simulink model "c00005M_harness"  (R2018a)
settings: Solver=ode3  StartTime=0.0  StopTime=10.0  RelTol=1e-3  EnableMultiTasking=on
undefined symbols (not defined in the file): b, DiscIntNeverNeededParam, J, K, L, PosMinimaW3, PosMinimaW4, R, sigbuilder_block
(part 3 of 9)

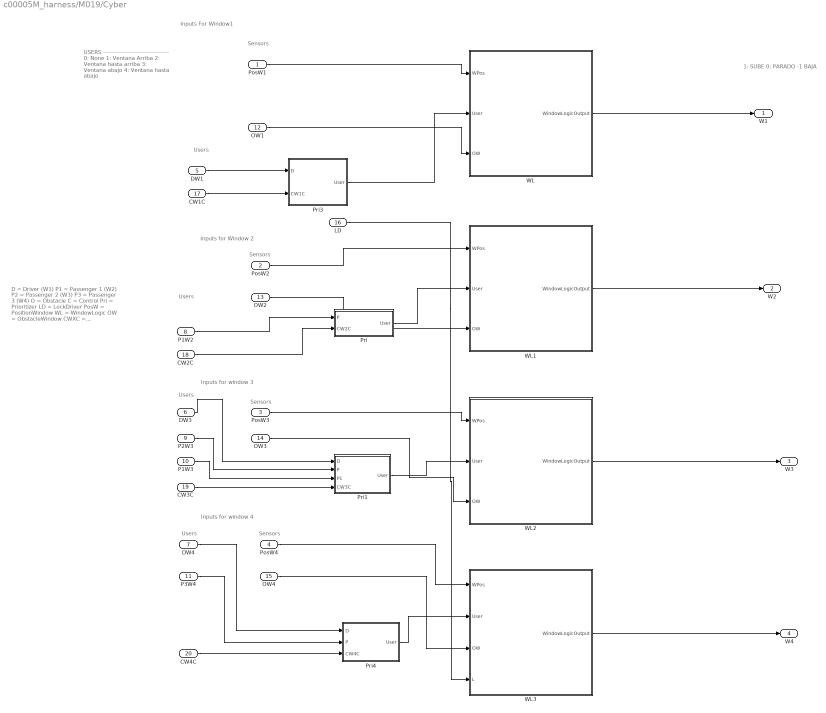
== system c00005M_harness/M019/Cyber ==
  note: Sensors
  note: Inputs For Window1
  note: Inputs for Window 2
  note: Inputs for window 3
  note: Inputs for window 4
  note: Users
  note: Users
  note: Sensors
  note: Users
  note: Sensors
  note: Users
  note: Sensors
  note: USERS
      | ---------------------------------
      | 0: None
      | 1: Ventana Arriba
      | 2: Ventana hasta arriba
      | 3: Ventana abajo
      | 4: Ventana hasta abajo
  note: 1: SUBE
      | 0: PARADO
      | -1 BAJA
  note: D = Driver (W1)
      | P1 = Passenger 1 (W2)
      | P2 = Passenger 2 (W3)
      | P3 = Passenger 3 (W4)
      | O = Obstacle
      | C = Control
      | Pri = Prioritizer
      | LD = LockDriver
      | PosW = PositionWindow
      | WL = WindowLogic
      | OW = ObstacleWindow
      | CWXC = ControlWindowXCentralized
      | S = Sensor
      | L = Lock
      | WPos = WindowPosition
      | M = Memory
      | InW = InputWindow
      | WIn = WindowInput
  PosW1 : Inport
  PosW2 : Inport  Port=2
  PosW3 : Inport  Port=3
  PosW4 : Inport  Port=4
  DW1 : Inport  Port=5
  DW3 : Inport  Port=6
  DW4 : Inport  Port=7
  P1W2 : Inport  Port=8
  P2W3 : Inport  Port=9
  P1W3 : Inport  Port=10
  P3W4 : Inport  Port=11
  OW1 : Inport  Port=12
  OW2 : Inport  Port=13
  OW3 : Inport  Port=14
  OW4 : Inport  Port=15
  LD : Inport  Port=16
  CW1C : Inport  Port=17
  CW2C : Inport  Port=18
  CW3C : Inport  Port=19
  CW4C : Inport  Port=20
  Pri : Subsystem
  Pri1 : Subsystem
  Pri3 : Subsystem
  Pri4 : Subsystem
  WL : Subsystem
  WL1 : Subsystem
  WL2 : Subsystem
  WL3 : Subsystem
  W1 : Outport
  W2 : Outport  Port=2
  W3 : Outport  Port=3
  W4 : Outport  Port=4
  wires:
  CW4C/1 -> Pri4/3(CW4C)
  CW3C/1 -> Pri1/4(CW3C)
  CW2C/1 -> Pri/2(CW2C)
  CW1C/1 -> Pri3/2(CW1C)
  Pri3/1(User) -> WL/2(User)
  WL3/1(WindowLogicOutput) -> W4/1
  WL2/1(WindowLogicOutput) -> W3/1
  Pri4/1(User) -> WL3/2(User)
  OW4/1 -> WL3/3(OW)
  PosW4/1 -> WL3/1(WPos)
  P3W4/1 -> Pri4/2(P)
  DW4/1 -> Pri4/1(D)
  P1W3/1 -> Pri1/3(P1)
  P2W3/1 -> Pri1/2(P)
  DW3/1 -> Pri1/1(D)
  OW3/1 -> WL2/3(OW)
  PosW3/1 -> WL2/1(WPos)
  Pri1/1(User) -> WL2/2(User)
  WL1/1(WindowLogicOutput) -> W2/1
  OW2/1 -> WL1/3(OW)
  PosW2/1 -> WL1/1(WPos)
  P1W2/1 -> Pri/1(P)
  Pri/1(User) -> WL1/2(User)
  WL/1(WindowLogicOutput) -> W1/1
  DW1/1 -> Pri3/1(D)
  OW1/1 -> WL/3(OW)
  PosW1/1 -> WL/1(WPos)
  LD/1 -> WL3/4(L)

== system c00005M_harness/M019/Physical ==
  InW1 : Inport
  InW2 : Inport  Port=2
  InW3 : Inport  Port=3
  InW4 : Inport  Port=4
  W : Subsystem
  W5 : Subsystem
  W6 : Subsystem
  W7 : Subsystem
  W1 : Outport
  W2 : Outport  Port=2
  W3 : Outport  Port=3
  W4 : Outport  Port=4
  wires:
  W7/1(WPos) -> W4/1
  W6/1(WPos) -> W3/1
  W5/1(WPos) -> W2/1
  W/1(WPos) -> W1/1
  InW4/1 -> W7/1(WIn)
  InW3/1 -> W6/1(WIn)
  InW2/1 -> W5/1(WIn)
  InW1/1 -> W/1(WIn)

== system c00005M_harness/M019/S1 ==
  PhyMeasure : Inport
  SensorOut : Outport
  wires:
  PhyMeasure/1 -> SensorOut/1

== system c00005M_harness/M019/S2 ==
  PhyMeasure : Inport
  SensorOut : Outport
  wires:
  PhyMeasure/1 -> SensorOut/1

== system c00005M_harness/M019/S3 ==
  PhyMeasure : Inport
  SensorOut : Outport
  wires:
  PhyMeasure/1 -> SensorOut/1

== system c00005M_harness/M019/S4 ==
  PhyMeasure : Inport
  SensorOut : Outport
  wires:
  PhyMeasure/1 -> SensorOut/1

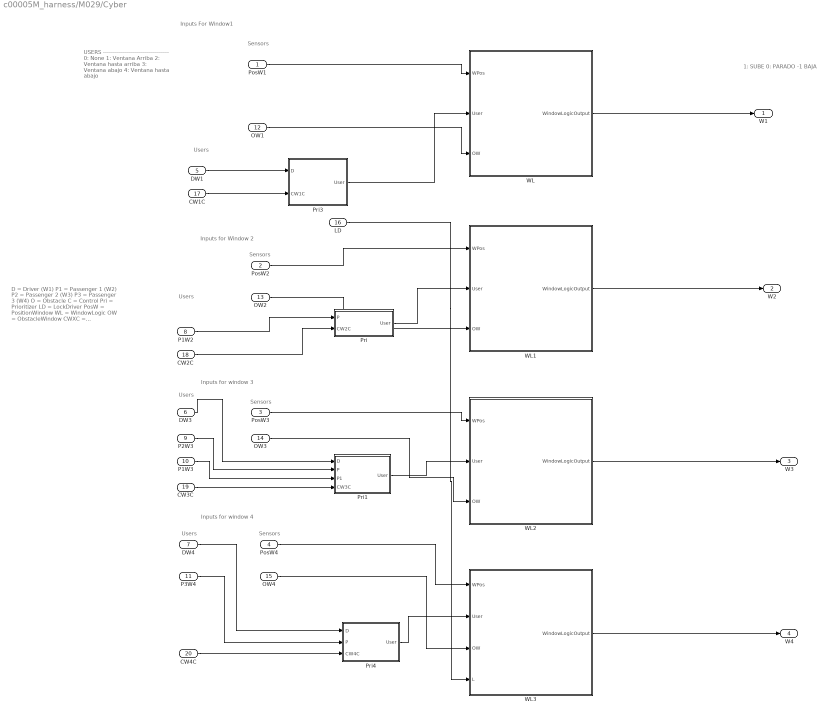
== system c00005M_harness/M029/Cyber ==
  note: Sensors
  note: Inputs For Window1
  note: Inputs for Window 2
  note: Inputs for window 3
  note: Inputs for window 4
  note: Users
  note: Users
  note: Sensors
  note: Users
  note: Sensors
  note: Users
  note: Sensors
  note: USERS
      | ---------------------------------
      | 0: None
      | 1: Ventana Arriba
      | 2: Ventana hasta arriba
      | 3: Ventana abajo
      | 4: Ventana hasta abajo
  note: 1: SUBE
      | 0: PARADO
      | -1 BAJA
  note: D = Driver (W1)
      | P1 = Passenger 1 (W2)
      | P2 = Passenger 2 (W3)
      | P3 = Passenger 3 (W4)
      | O = Obstacle
      | C = Control
      | Pri = Prioritizer
      | LD = LockDriver
      | PosW = PositionWindow
      | WL = WindowLogic
      | OW = ObstacleWindow
      | CWXC = ControlWindowXCentralized
      | S = Sensor
      | L = Lock
      | WPos = WindowPosition
      | M = Memory
      | InW = InputWindow
      | WIn = WindowInput
  PosW1 : Inport
  PosW2 : Inport  Port=2
  PosW3 : Inport  Port=3
  PosW4 : Inport  Port=4
  DW1 : Inport  Port=5
  DW3 : Inport  Port=6
  DW4 : Inport  Port=7
  P1W2 : Inport  Port=8
  P2W3 : Inport  Port=9
  P1W3 : Inport  Port=10
  P3W4 : Inport  Port=11
  OW1 : Inport  Port=12
  OW2 : Inport  Port=13
  OW3 : Inport  Port=14
  OW4 : Inport  Port=15
  LD : Inport  Port=16
  CW1C : Inport  Port=17
  CW2C : Inport  Port=18
  CW3C : Inport  Port=19
  CW4C : Inport  Port=20
  Pri : Subsystem
  Pri1 : Subsystem
  Pri3 : Subsystem
  Pri4 : Subsystem
  WL : Subsystem
  WL1 : Subsystem
  WL2 : Subsystem
  WL3 : Subsystem
  W1 : Outport
  W2 : Outport  Port=2
  W3 : Outport  Port=3
  W4 : Outport  Port=4
  wires:
  CW4C/1 -> Pri4/3(CW4C)
  CW3C/1 -> Pri1/4(CW3C)
  CW2C/1 -> Pri/2(CW2C)
  CW1C/1 -> Pri3/2(CW1C)
  Pri3/1(User) -> WL/2(User)
  WL3/1(WindowLogicOutput) -> W4/1
  WL2/1(WindowLogicOutput) -> W3/1
  Pri4/1(User) -> WL3/2(User)
  OW4/1 -> WL3/3(OW)
  PosW4/1 -> WL3/1(WPos)
  P3W4/1 -> Pri4/2(P)
  DW4/1 -> Pri4/1(D)
  P1W3/1 -> Pri1/3(P1)
  P2W3/1 -> Pri1/2(P)
  DW3/1 -> Pri1/1(D)
  OW3/1 -> WL2/3(OW)
  PosW3/1 -> WL2/1(WPos)
  Pri1/1(User) -> WL2/2(User)
  WL1/1(WindowLogicOutput) -> W2/1
  OW2/1 -> WL1/3(OW)
  PosW2/1 -> WL1/1(WPos)
  P1W2/1 -> Pri/1(P)
  Pri/1(User) -> WL1/2(User)
  WL/1(WindowLogicOutput) -> W1/1
  DW1/1 -> Pri3/1(D)
  OW1/1 -> WL/3(OW)
  PosW1/1 -> WL/1(WPos)
  LD/1 -> WL3/4(L)

== system c00005M_harness/M029/Physical ==
  InW1 : Inport
  InW2 : Inport  Port=2
  InW3 : Inport  Port=3
  InW4 : Inport  Port=4
  W : Subsystem
  W5 : Subsystem
  W6 : Subsystem
  W7 : Subsystem
  W1 : Outport
  W2 : Outport  Port=2
  W3 : Outport  Port=3
  W4 : Outport  Port=4
  wires:
  W7/1(WPos) -> W4/1
  W6/1(WPos) -> W3/1
  W5/1(WPos) -> W2/1
  W/1(WPos) -> W1/1
  InW4/1 -> W7/1(WIn)
  InW3/1 -> W6/1(WIn)
  InW2/1 -> W5/1(WIn)
  InW1/1 -> W/1(WIn)

== system c00005M_harness/M029/S1 ==
  PhyMeasure : Inport
  SensorOut : Outport
  wires:
  PhyMeasure/1 -> SensorOut/1

== system c00005M_harness/M029/S2 ==
  PhyMeasure : Inport
  SensorOut : Outport
  wires:
  PhyMeasure/1 -> SensorOut/1

== system c00005M_harness/M029/S3 ==
  PhyMeasure : Inport
  SensorOut : Outport
  wires:
  PhyMeasure/1 -> SensorOut/1

== system c00005M_harness/M029/S4 ==
  PhyMeasure : Inport
  SensorOut : Outport
  wires:
  PhyMeasure/1 -> SensorOut/1

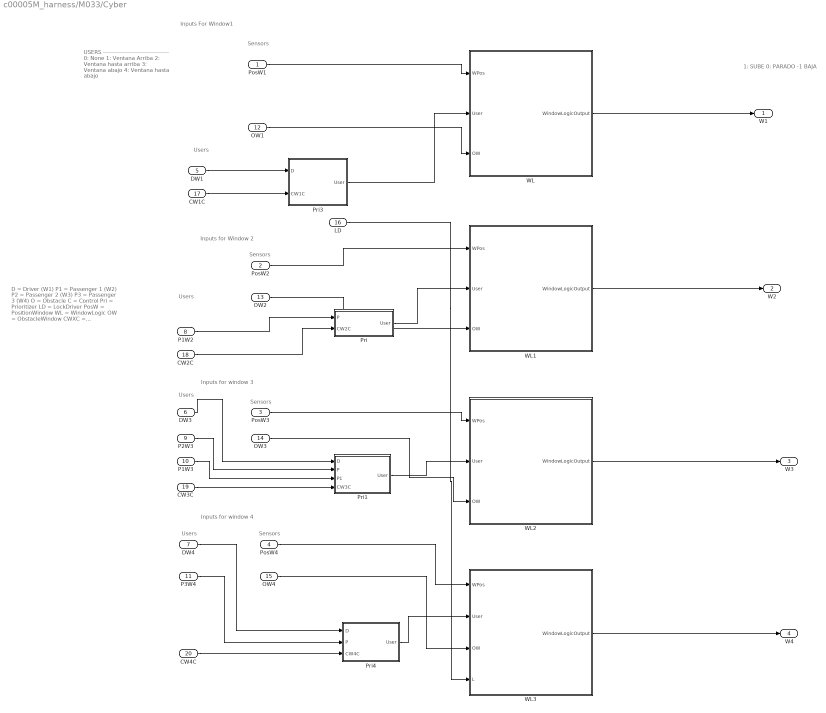
== system c00005M_harness/M033/Cyber ==
  note: Sensors
  note: Inputs For Window1
  note: Inputs for Window 2
  note: Inputs for window 3
  note: Inputs for window 4
  note: Users
  note: Users
  note: Sensors
  note: Users
  note: Sensors
  note: Users
  note: Sensors
  note: USERS
      | ---------------------------------
      | 0: None
      | 1: Ventana Arriba
      | 2: Ventana hasta arriba
      | 3: Ventana abajo
      | 4: Ventana hasta abajo
  note: 1: SUBE
      | 0: PARADO
      | -1 BAJA
  note: D = Driver (W1)
      | P1 = Passenger 1 (W2)
      | P2 = Passenger 2 (W3)
      | P3 = Passenger 3 (W4)
      | O = Obstacle
      | C = Control
      | Pri = Prioritizer
      | LD = LockDriver
      | PosW = PositionWindow
      | WL = WindowLogic
      | OW = ObstacleWindow
      | CWXC = ControlWindowXCentralized
      | S = Sensor
      | L = Lock
      | WPos = WindowPosition
      | M = Memory
      | InW = InputWindow
      | WIn = WindowInput
  PosW1 : Inport
  PosW2 : Inport  Port=2
  PosW3 : Inport  Port=3
  PosW4 : Inport  Port=4
  DW1 : Inport  Port=5
  DW3 : Inport  Port=6
  DW4 : Inport  Port=7
  P1W2 : Inport  Port=8
  P2W3 : Inport  Port=9
  P1W3 : Inport  Port=10
  P3W4 : Inport  Port=11
  OW1 : Inport  Port=12
  OW2 : Inport  Port=13
  OW3 : Inport  Port=14
  OW4 : Inport  Port=15
  LD : Inport  Port=16
  CW1C : Inport  Port=17
  CW2C : Inport  Port=18
  CW3C : Inport  Port=19
  CW4C : Inport  Port=20
  Pri : Subsystem
  Pri1 : Subsystem
  Pri3 : Subsystem
  Pri4 : Subsystem
  WL : Subsystem
  WL1 : Subsystem
  WL2 : Subsystem
  WL3 : Subsystem
  W1 : Outport
  W2 : Outport  Port=2
  W3 : Outport  Port=3
  W4 : Outport  Port=4
  wires:
  CW4C/1 -> Pri4/3(CW4C)
  CW3C/1 -> Pri1/4(CW3C)
  CW2C/1 -> Pri/2(CW2C)
  CW1C/1 -> Pri3/2(CW1C)
  Pri3/1(User) -> WL/2(User)
  WL3/1(WindowLogicOutput) -> W4/1
  WL2/1(WindowLogicOutput) -> W3/1
  Pri4/1(User) -> WL3/2(User)
  OW4/1 -> WL3/3(OW)
  PosW4/1 -> WL3/1(WPos)
  P3W4/1 -> Pri4/2(P)
  DW4/1 -> Pri4/1(D)
  P1W3/1 -> Pri1/3(P1)
  P2W3/1 -> Pri1/2(P)
  DW3/1 -> Pri1/1(D)
  OW3/1 -> WL2/3(OW)
  PosW3/1 -> WL2/1(WPos)
  Pri1/1(User) -> WL2/2(User)
  WL1/1(WindowLogicOutput) -> W2/1
  OW2/1 -> WL1/3(OW)
  PosW2/1 -> WL1/1(WPos)
  P1W2/1 -> Pri/1(P)
  Pri/1(User) -> WL1/2(User)
  WL/1(WindowLogicOutput) -> W1/1
  DW1/1 -> Pri3/1(D)
  OW1/1 -> WL/3(OW)
  PosW1/1 -> WL/1(WPos)
  LD/1 -> WL3/4(L)

== system c00005M_harness/M033/Physical ==
  InW1 : Inport
  InW2 : Inport  Port=2
  InW3 : Inport  Port=3
  InW4 : Inport  Port=4
  W : Subsystem
  W5 : Subsystem
  W6 : Subsystem
  W7 : Subsystem
  W1 : Outport
  W2 : Outport  Port=2
  W3 : Outport  Port=3
  W4 : Outport  Port=4
  wires:
  W7/1(WPos) -> W4/1
  W6/1(WPos) -> W3/1
  W5/1(WPos) -> W2/1
  W/1(WPos) -> W1/1
  InW4/1 -> W7/1(WIn)
  InW3/1 -> W6/1(WIn)
  InW2/1 -> W5/1(WIn)
  InW1/1 -> W/1(WIn)

== system c00005M_harness/M033/S1 ==
  PhyMeasure : Inport
  SensorOut : Outport
  wires:
  PhyMeasure/1 -> SensorOut/1

== system c00005M_harness/M033/S2 ==
  PhyMeasure : Inport
  SensorOut : Outport
  wires:
  PhyMeasure/1 -> SensorOut/1

== system c00005M_harness/M033/S3 ==
  PhyMeasure : Inport
  SensorOut : Outport
  wires:
  PhyMeasure/1 -> SensorOut/1

== system c00005M_harness/M033/S4 ==
  PhyMeasure : Inport
  SensorOut : Outport
  wires:
  PhyMeasure/1 -> SensorOut/1

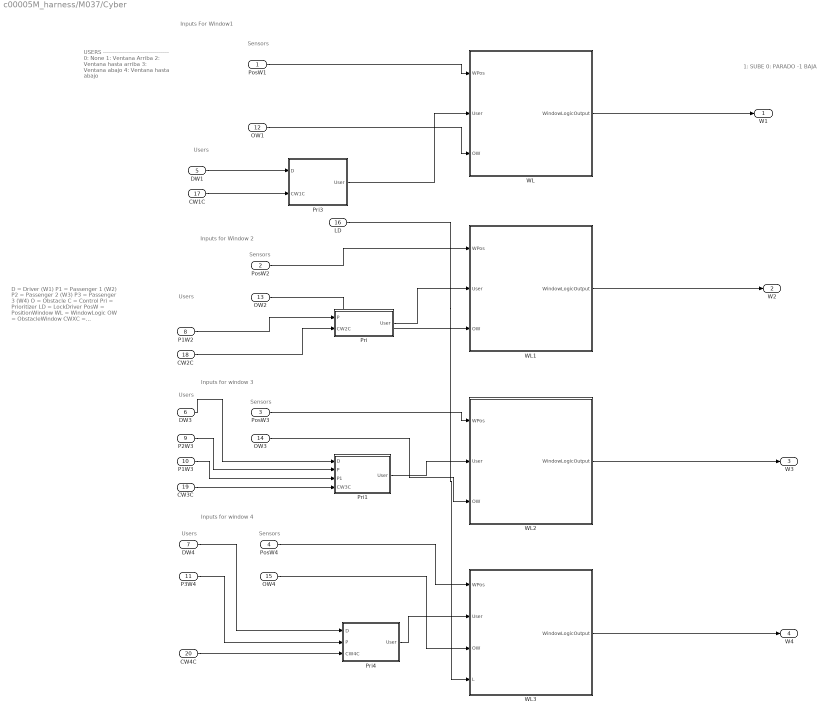
== system c00005M_harness/M037/Cyber ==
  note: Sensors
  note: Inputs For Window1
  note: Inputs for Window 2
  note: Inputs for window 3
  note: Inputs for window 4
  note: Users
  note: Users
  note: Sensors
  note: Users
  note: Sensors
  note: Users
  note: Sensors
  note: USERS
      | ---------------------------------
      | 0: None
      | 1: Ventana Arriba
      | 2: Ventana hasta arriba
      | 3: Ventana abajo
      | 4: Ventana hasta abajo
  note: 1: SUBE
      | 0: PARADO
      | -1 BAJA
  note: D = Driver (W1)
      | P1 = Passenger 1 (W2)
      | P2 = Passenger 2 (W3)
      | P3 = Passenger 3 (W4)
      | O = Obstacle
      | C = Control
      | Pri = Prioritizer
      | LD = LockDriver
      | PosW = PositionWindow
      | WL = WindowLogic
      | OW = ObstacleWindow
      | CWXC = ControlWindowXCentralized
      | S = Sensor
      | L = Lock
      | WPos = WindowPosition
      | M = Memory
      | InW = InputWindow
      | WIn = WindowInput
  PosW1 : Inport
  PosW2 : Inport  Port=2
  PosW3 : Inport  Port=3
  PosW4 : Inport  Port=4
  DW1 : Inport  Port=5
  DW3 : Inport  Port=6
  DW4 : Inport  Port=7
  P1W2 : Inport  Port=8
  P2W3 : Inport  Port=9
  P1W3 : Inport  Port=10
  P3W4 : Inport  Port=11
  OW1 : Inport  Port=12
  OW2 : Inport  Port=13
  OW3 : Inport  Port=14
  OW4 : Inport  Port=15
  LD : Inport  Port=16
  CW1C : Inport  Port=17
  CW2C : Inport  Port=18
  CW3C : Inport  Port=19
  CW4C : Inport  Port=20
  Pri : Subsystem
  Pri1 : Subsystem
  Pri3 : Subsystem
  Pri4 : Subsystem
  WL : Subsystem
  WL1 : Subsystem
  WL2 : Subsystem
  WL3 : Subsystem
  W1 : Outport
  W2 : Outport  Port=2
  W3 : Outport  Port=3
  W4 : Outport  Port=4
  wires:
  CW4C/1 -> Pri4/3(CW4C)
  CW3C/1 -> Pri1/4(CW3C)
  CW2C/1 -> Pri/2(CW2C)
  CW1C/1 -> Pri3/2(CW1C)
  Pri3/1(User) -> WL/2(User)
  WL3/1(WindowLogicOutput) -> W4/1
  WL2/1(WindowLogicOutput) -> W3/1
  Pri4/1(User) -> WL3/2(User)
  OW4/1 -> WL3/3(OW)
  PosW4/1 -> WL3/1(WPos)
  P3W4/1 -> Pri4/2(P)
  DW4/1 -> Pri4/1(D)
  P1W3/1 -> Pri1/3(P1)
  P2W3/1 -> Pri1/2(P)
  DW3/1 -> Pri1/1(D)
  OW3/1 -> WL2/3(OW)
  PosW3/1 -> WL2/1(WPos)
  Pri1/1(User) -> WL2/2(User)
  WL1/1(WindowLogicOutput) -> W2/1
  OW2/1 -> WL1/3(OW)
  PosW2/1 -> WL1/1(WPos)
  P1W2/1 -> Pri/1(P)
  Pri/1(User) -> WL1/2(User)
  WL/1(WindowLogicOutput) -> W1/1
  DW1/1 -> Pri3/1(D)
  OW1/1 -> WL/3(OW)
  PosW1/1 -> WL/1(WPos)
  LD/1 -> WL3/4(L)

== system c00005M_harness/M037/Physical ==
  InW1 : Inport
  InW2 : Inport  Port=2
  InW3 : Inport  Port=3
  InW4 : Inport  Port=4
  W : Subsystem
  W5 : Subsystem
  W6 : Subsystem
  W7 : Subsystem
  W1 : Outport
  W2 : Outport  Port=2
  W3 : Outport  Port=3
  W4 : Outport  Port=4
  wires:
  W7/1(WPos) -> W4/1
  W6/1(WPos) -> W3/1
  W5/1(WPos) -> W2/1
  W/1(WPos) -> W1/1
  InW4/1 -> W7/1(WIn)
  InW3/1 -> W6/1(WIn)
  InW2/1 -> W5/1(WIn)
  InW1/1 -> W/1(WIn)

== system c00005M_harness/M037/S1 ==
  PhyMeasure : Inport
  SensorOut : Outport
  wires:
  PhyMeasure/1 -> SensorOut/1

== system c00005M_harness/M037/S2 ==
  PhyMeasure : Inport
  SensorOut : Outport
  wires:
  PhyMeasure/1 -> SensorOut/1

== system c00005M_harness/M037/S3 ==
  PhyMeasure : Inport
  SensorOut : Outport
  wires:
  PhyMeasure/1 -> SensorOut/1

== system c00005M_harness/M037/S4 ==
  PhyMeasure : Inport
  SensorOut : Outport
  wires:
  PhyMeasure/1 -> SensorOut/1

== system c00005M_harness/M040/Cyber ==
  note: Sensors
  note: Inputs For Window1
  note: Inputs for Window 2
  note: Inputs for window 3
  note: Inputs for window 4
  note: Users
  note: Users
  note: Sensors
  note: Users
  note: Sensors
  note: Users
  note: Sensors
  note: USERS
      | ---------------------------------
      | 0: None
      | 1: Ventana Arriba
      | 2: Ventana hasta arriba
      | 3: Ventana abajo
      | 4: Ventana hasta abajo
  note: 1: SUBE
      | 0: PARADO
      | -1 BAJA
  note: D = Driver (W1)
      | P1 = Passenger 1 (W2)
      | P2 = Passenger 2 (W3)
      | P3 = Passenger 3 (W4)
      | O = Obstacle
      | C = Control
      | Pri = Prioritizer
      | LD = LockDriver
      | PosW = PositionWindow
      | WL = WindowLogic
      | OW = ObstacleWindow
      | CWXC = ControlWindowXCentralized
      | S = Sensor
      | L = Lock
      | WPos = WindowPosition
      | M = Memory
      | InW = InputWindow
      | WIn = WindowInput
  PosW1 : Inport
  PosW2 : Inport  Port=2
  PosW3 : Inport  Port=3
  PosW4 : Inport  Port=4
  DW1 : Inport  Port=5
  DW3 : Inport  Port=6
  DW4 : Inport  Port=7
  P1W2 : Inport  Port=8
  P2W3 : Inport  Port=9
  P1W3 : Inport  Port=10
  P3W4 : Inport  Port=11
  OW1 : Inport  Port=12
  OW2 : Inport  Port=13
  OW3 : Inport  Port=14
  OW4 : Inport  Port=15
  LD : Inport  Port=16
  CW1C : Inport  Port=17
  CW2C : Inport  Port=18
  CW3C : Inport  Port=19
  CW4C : Inport  Port=20
  Pri : Subsystem
  Pri1 : Subsystem
  Pri3 : Subsystem
  Pri4 : Subsystem
  WL : Subsystem
  WL1 : Subsystem
  WL2 : Subsystem
  WL3 : Subsystem
  W1 : Outport
  W2 : Outport  Port=2
  W3 : Outport  Port=3
  W4 : Outport  Port=4
  wires:
  CW4C/1 -> Pri4/3(CW4C)
  CW3C/1 -> Pri1/4(CW3C)
  CW2C/1 -> Pri/2(CW2C)
  CW1C/1 -> Pri3/2(CW1C)
  Pri3/1(User) -> WL/2(User)
  WL3/1(WindowLogicOutput) -> W4/1
  WL2/1(WindowLogicOutput) -> W3/1
  Pri4/1(User) -> WL3/2(User)
  OW4/1 -> WL3/3(OW)
  PosW4/1 -> WL3/1(WPos)
  P3W4/1 -> Pri4/2(P)
  DW4/1 -> Pri4/1(D)
  P1W3/1 -> Pri1/3(P1)
  P2W3/1 -> Pri1/2(P)
  DW3/1 -> Pri1/1(D)
  OW3/1 -> WL2/3(OW)
  PosW3/1 -> WL2/1(WPos)
  Pri1/1(User) -> WL2/2(User)
  WL1/1(WindowLogicOutput) -> W2/1
  OW2/1 -> WL1/3(OW)
  PosW2/1 -> WL1/1(WPos)
  P1W2/1 -> Pri/1(P)
  Pri/1(User) -> WL1/2(User)
  WL/1(WindowLogicOutput) -> W1/1
  DW1/1 -> Pri3/1(D)
  OW1/1 -> WL/3(OW)
  PosW1/1 -> WL/1(WPos)
  LD/1 -> WL3/4(L)

== system c00005M_harness/M040/Physical ==
  InW1 : Inport
  InW2 : Inport  Port=2
  InW3 : Inport  Port=3
  InW4 : Inport  Port=4
  W : Subsystem
  W5 : Subsystem
  W6 : Subsystem
  W7 : Subsystem
  W1 : Outport
  W2 : Outport  Port=2
  W3 : Outport  Port=3
  W4 : Outport  Port=4
  wires:
  W7/1(WPos) -> W4/1
  W6/1(WPos) -> W3/1
  W5/1(WPos) -> W2/1
  W/1(WPos) -> W1/1
  InW4/1 -> W7/1(WIn)
  InW3/1 -> W6/1(WIn)
  InW2/1 -> W5/1(WIn)
  InW1/1 -> W/1(WIn)

== system c00005M_harness/M040/S1 ==
  PhyMeasure : Inport
  SensorOut : Outport
  wires:
  PhyMeasure/1 -> SensorOut/1

== system c00005M_harness/M040/S2 ==
  PhyMeasure : Inport
  SensorOut : Outport
  wires:
  PhyMeasure/1 -> SensorOut/1

== system c00005M_harness/M040/S3 ==
  PhyMeasure : Inport
  SensorOut : Outport
  wires:
  PhyMeasure/1 -> SensorOut/1

== system c00005M_harness/M040/S4 ==
  PhyMeasure : Inport
  SensorOut : Outport
  wires:
  PhyMeasure/1 -> SensorOut/1

== system c00005M_harness/M041/Cyber ==
  note: Sensors
  note: Inputs For Window1
  note: Inputs for Window 2
  note: Inputs for window 3
  note: Inputs for window 4
  note: Users
  note: Users
  note: Sensors
  note: Users
  note: Sensors
  note: Users
  note: Sensors
  note: USERS
      | ---------------------------------
      | 0: None
      | 1: Ventana Arriba
      | 2: Ventana hasta arriba
      | 3: Ventana abajo
      | 4: Ventana hasta abajo
  note: 1: SUBE
      | 0: PARADO
      | -1 BAJA
  note: D = Driver (W1)
      | P1 = Passenger 1 (W2)
      | P2 = Passenger 2 (W3)
      | P3 = Passenger 3 (W4)
      | O = Obstacle
      | C = Control
      | Pri = Prioritizer
      | LD = LockDriver
      | PosW = PositionWindow
      | WL = WindowLogic
      | OW = ObstacleWindow
      | CWXC = ControlWindowXCentralized
      | S = Sensor
      | L = Lock
      | WPos = WindowPosition
      | M = Memory
      | InW = InputWindow
      | WIn = WindowInput
  PosW1 : Inport
  PosW2 : Inport  Port=2
  PosW3 : Inport  Port=3
  PosW4 : Inport  Port=4
  DW1 : Inport  Port=5
  DW3 : Inport  Port=6
  DW4 : Inport  Port=7
  P1W2 : Inport  Port=8
  P2W3 : Inport  Port=9
  P1W3 : Inport  Port=10
  P3W4 : Inport  Port=11
  OW1 : Inport  Port=12
  OW2 : Inport  Port=13
  OW3 : Inport  Port=14
  OW4 : Inport  Port=15
  LD : Inport  Port=16
  CW1C : Inport  Port=17
  CW2C : Inport  Port=18
  CW3C : Inport  Port=19
  CW4C : Inport  Port=20
  Pri : Subsystem
  Pri1 : Subsystem
  Pri3 : Subsystem
  Pri4 : Subsystem
  WL : Subsystem
  WL1 : Subsystem
  WL2 : Subsystem
  WL3 : Subsystem
  W1 : Outport
  W2 : Outport  Port=2
  W3 : Outport  Port=3
  W4 : Outport  Port=4
  wires:
  CW4C/1 -> Pri4/3(CW4C)
  CW3C/1 -> Pri1/4(CW3C)
  CW2C/1 -> Pri/2(CW2C)
  CW1C/1 -> Pri3/2(CW1C)
  Pri3/1(User) -> WL/2(User)
  WL3/1(WindowLogicOutput) -> W4/1
  WL2/1(WindowLogicOutput) -> W3/1
  Pri4/1(User) -> WL3/2(User)
  OW4/1 -> WL3/3(OW)
  PosW4/1 -> WL3/1(WPos)
  P3W4/1 -> Pri4/2(P)
  DW4/1 -> Pri4/1(D)
  P1W3/1 -> Pri1/3(P1)
  P2W3/1 -> Pri1/2(P)
  DW3/1 -> Pri1/1(D)
  OW3/1 -> WL2/3(OW)
  PosW3/1 -> WL2/1(WPos)
  Pri1/1(User) -> WL2/2(User)
  WL1/1(WindowLogicOutput) -> W2/1
  OW2/1 -> WL1/3(OW)
  PosW2/1 -> WL1/1(WPos)
  P1W2/1 -> Pri/1(P)
  Pri/1(User) -> WL1/2(User)
  WL/1(WindowLogicOutput) -> W1/1
  DW1/1 -> Pri3/1(D)
  OW1/1 -> WL/3(OW)
  PosW1/1 -> WL/1(WPos)
  LD/1 -> WL3/4(L)

== system c00005M_harness/M041/Physical ==
  InW1 : Inport
  InW2 : Inport  Port=2
  InW3 : Inport  Port=3
  InW4 : Inport  Port=4
  W : Subsystem
  W5 : Subsystem
  W6 : Subsystem
  W7 : Subsystem
  W1 : Outport
  W2 : Outport  Port=2
  W3 : Outport  Port=3
  W4 : Outport  Port=4
  wires:
  W7/1(WPos) -> W4/1
  W6/1(WPos) -> W3/1
  W5/1(WPos) -> W2/1
  W/1(WPos) -> W1/1
  InW4/1 -> W7/1(WIn)
  InW3/1 -> W6/1(WIn)
  InW2/1 -> W5/1(WIn)
  InW1/1 -> W/1(WIn)

== system c00005M_harness/M041/S1 ==
  PhyMeasure : Inport
  SensorOut : Outport
  wires:
  PhyMeasure/1 -> SensorOut/1

== system c00005M_harness/M041/S2 ==
  PhyMeasure : Inport
  SensorOut : Outport
  wires:
  PhyMeasure/1 -> SensorOut/1

== system c00005M_harness/M041/S3 ==
  PhyMeasure : Inport
  SensorOut : Outport
  wires:
  PhyMeasure/1 -> SensorOut/1

== system c00005M_harness/M041/S4 ==
  PhyMeasure : Inport
  SensorOut : Outport
  wires:
  PhyMeasure/1 -> SensorOut/1

== system c00005M_harness/M043/Cyber ==
  note: Sensors
  note: Inputs For Window1
  note: Inputs for Window 2
  note: Inputs for window 3
  note: Inputs for window 4
  note: Users
  note: Users
  note: Sensors
  note: Users
  note: Sensors
  note: Users
  note: Sensors
  note: USERS
      | ---------------------------------
      | 0: None
      | 1: Ventana Arriba
      | 2: Ventana hasta arriba
      | 3: Ventana abajo
      | 4: Ventana hasta abajo
  note: 1: SUBE
      | 0: PARADO
      | -1 BAJA
  note: D = Driver (W1)
      | P1 = Passenger 1 (W2)
      | P2 = Passenger 2 (W3)
      | P3 = Passenger 3 (W4)
      | O = Obstacle
      | C = Control
      | Pri = Prioritizer
      | LD = LockDriver
      | PosW = PositionWindow
      | WL = WindowLogic
      | OW = ObstacleWindow
      | CWXC = ControlWindowXCentralized
      | S = Sensor
      | L = Lock
      | WPos = WindowPosition
      | M = Memory
      | InW = InputWindow
      | WIn = WindowInput
  PosW1 : Inport
  PosW2 : Inport  Port=2
  PosW3 : Inport  Port=3
  PosW4 : Inport  Port=4
  DW1 : Inport  Port=5
  DW3 : Inport  Port=6
  DW4 : Inport  Port=7
  P1W2 : Inport  Port=8
  P2W3 : Inport  Port=9
  P1W3 : Inport  Port=10
  P3W4 : Inport  Port=11
  OW1 : Inport  Port=12
  OW2 : Inport  Port=13
  OW3 : Inport  Port=14
  OW4 : Inport  Port=15
  LD : Inport  Port=16
  CW1C : Inport  Port=17
  CW2C : Inport  Port=18
  CW3C : Inport  Port=19
  CW4C : Inport  Port=20
  Pri : Subsystem
  Pri1 : Subsystem
  Pri3 : Subsystem
  Pri4 : Subsystem
  WL : Subsystem
  WL1 : Subsystem
  WL2 : Subsystem
  WL3 : Subsystem
  W1 : Outport
  W2 : Outport  Port=2
  W3 : Outport  Port=3
  W4 : Outport  Port=4
  wires:
  CW4C/1 -> Pri4/3(CW4C)
  CW3C/1 -> Pri1/4(CW3C)
  CW2C/1 -> Pri/2(CW2C)
  CW1C/1 -> Pri3/2(CW1C)
  Pri3/1(User) -> WL/2(User)
  WL3/1(WindowLogicOutput) -> W4/1
  WL2/1(WindowLogicOutput) -> W3/1
  Pri4/1(User) -> WL3/2(User)
  OW4/1 -> WL3/3(OW)
  PosW4/1 -> WL3/1(WPos)
  P3W4/1 -> Pri4/2(P)
  DW4/1 -> Pri4/1(D)
  P1W3/1 -> Pri1/3(P1)
  P2W3/1 -> Pri1/2(P)
  DW3/1 -> Pri1/1(D)
  OW3/1 -> WL2/3(OW)
  PosW3/1 -> WL2/1(WPos)
  Pri1/1(User) -> WL2/2(User)
  WL1/1(WindowLogicOutput) -> W2/1
  OW2/1 -> WL1/3(OW)
  PosW2/1 -> WL1/1(WPos)
  P1W2/1 -> Pri/1(P)
  Pri/1(User) -> WL1/2(User)
  WL/1(WindowLogicOutput) -> W1/1
  DW1/1 -> Pri3/1(D)
  OW1/1 -> WL/3(OW)
  PosW1/1 -> WL/1(WPos)
  LD/1 -> WL3/4(L)

== system c00005M_harness/M043/Physical ==
  InW1 : Inport
  InW2 : Inport  Port=2
  InW3 : Inport  Port=3
  InW4 : Inport  Port=4
  W : Subsystem
  W5 : Subsystem
  W6 : Subsystem
  W7 : Subsystem
  W1 : Outport
  W2 : Outport  Port=2
  W3 : Outport  Port=3
  W4 : Outport  Port=4
  wires:
  W7/1(WPos) -> W4/1
  W6/1(WPos) -> W3/1
  W5/1(WPos) -> W2/1
  W/1(WPos) -> W1/1
  InW4/1 -> W7/1(WIn)
  InW3/1 -> W6/1(WIn)
  InW2/1 -> W5/1(WIn)
  InW1/1 -> W/1(WIn)

== system c00005M_harness/M043/S1 ==
  PhyMeasure : Inport
  SensorOut : Outport
  wires:
  PhyMeasure/1 -> SensorOut/1

== system c00005M_harness/M043/S2 ==
  PhyMeasure : Inport
  SensorOut : Outport
  wires:
  PhyMeasure/1 -> SensorOut/1

== system c00005M_harness/M043/S3 ==
  PhyMeasure : Inport
  SensorOut : Outport
  wires:
  PhyMeasure/1 -> SensorOut/1

== system c00005M_harness/M043/S4 ==
  PhyMeasure : Inport
  SensorOut : Outport
  wires:
  PhyMeasure/1 -> SensorOut/1

== system c00005M_harness/M046/Cyber ==
  note: Sensors
  note: Inputs For Window1
  note: Inputs for Window 2
  note: Inputs for window 3
  note: Inputs for window 4
  note: Users
  note: Users
  note: Sensors
  note: Users
  note: Sensors
  note: Users
  note: Sensors
  note: USERS
      | ---------------------------------
      | 0: None
      | 1: Ventana Arriba
      | 2: Ventana hasta arriba
      | 3: Ventana abajo
      | 4: Ventana hasta abajo
  note: 1: SUBE
      | 0: PARADO
      | -1 BAJA
  note: D = Driver (W1)
      | P1 = Passenger 1 (W2)
      | P2 = Passenger 2 (W3)
      | P3 = Passenger 3 (W4)
      | O = Obstacle
      | C = Control
      | Pri = Prioritizer
      | LD = LockDriver
      | PosW = PositionWindow
      | WL = WindowLogic
      | OW = ObstacleWindow
      | CWXC = ControlWindowXCentralized
      | S = Sensor
      | L = Lock
      | WPos = WindowPosition
      | M = Memory
      | InW = InputWindow
      | WIn = WindowInput
  PosW1 : Inport
  PosW2 : Inport  Port=2
  PosW3 : Inport  Port=3
  PosW4 : Inport  Port=4
  DW1 : Inport  Port=5
  DW3 : Inport  Port=6
  DW4 : Inport  Port=7
  P1W2 : Inport  Port=8
  P2W3 : Inport  Port=9
  P1W3 : Inport  Port=10
  P3W4 : Inport  Port=11
  OW1 : Inport  Port=12
  OW2 : Inport  Port=13
  OW3 : Inport  Port=14
  OW4 : Inport  Port=15
  LD : Inport  Port=16
  CW1C : Inport  Port=17
  CW2C : Inport  Port=18
  CW3C : Inport  Port=19
  CW4C : Inport  Port=20
  Pri : Subsystem
  Pri1 : Subsystem
  Pri3 : Subsystem
  Pri4 : Subsystem
  WL : Subsystem
  WL1 : Subsystem
  WL2 : Subsystem
  WL3 : Subsystem
  W1 : Outport
  W2 : Outport  Port=2
  W3 : Outport  Port=3
  W4 : Outport  Port=4
  wires:
  CW4C/1 -> Pri4/3(CW4C)
  CW3C/1 -> Pri1/4(CW3C)
  CW2C/1 -> Pri/2(CW2C)
  CW1C/1 -> Pri3/2(CW1C)
  Pri3/1(User) -> WL/2(User)
  WL3/1(WindowLogicOutput) -> W4/1
  WL2/1(WindowLogicOutput) -> W3/1
  Pri4/1(User) -> WL3/2(User)
  OW4/1 -> WL3/3(OW)
  PosW4/1 -> WL3/1(WPos)
  P3W4/1 -> Pri4/2(P)
  DW4/1 -> Pri4/1(D)
  P1W3/1 -> Pri1/3(P1)
  P2W3/1 -> Pri1/2(P)
  DW3/1 -> Pri1/1(D)
  OW3/1 -> WL2/3(OW)
  PosW3/1 -> WL2/1(WPos)
  Pri1/1(User) -> WL2/2(User)
  WL1/1(WindowLogicOutput) -> W2/1
  OW2/1 -> WL1/3(OW)
  PosW2/1 -> WL1/1(WPos)
  P1W2/1 -> Pri/1(P)
  Pri/1(User) -> WL1/2(User)
  WL/1(WindowLogicOutput) -> W1/1
  DW1/1 -> Pri3/1(D)
  OW1/1 -> WL/3(OW)
  PosW1/1 -> WL/1(WPos)
  LD/1 -> WL3/4(L)

== system c00005M_harness/M046/Physical ==
  InW1 : Inport
  InW2 : Inport  Port=2
  InW3 : Inport  Port=3
  InW4 : Inport  Port=4
  W : Subsystem
  W5 : Subsystem
  W6 : Subsystem
  W7 : Subsystem
  W1 : Outport
  W2 : Outport  Port=2
  W3 : Outport  Port=3
  W4 : Outport  Port=4
  wires:
  W7/1(WPos) -> W4/1
  W6/1(WPos) -> W3/1
  W5/1(WPos) -> W2/1
  W/1(WPos) -> W1/1
  InW4/1 -> W7/1(WIn)
  InW3/1 -> W6/1(WIn)
  InW2/1 -> W5/1(WIn)
  InW1/1 -> W/1(WIn)

== system c00005M_harness/M046/S1 ==
  PhyMeasure : Inport
  SensorOut : Outport
  wires:
  PhyMeasure/1 -> SensorOut/1

== system c00005M_harness/M046/S2 ==
  PhyMeasure : Inport
  SensorOut : Outport
  wires:
  PhyMeasure/1 -> SensorOut/1

== system c00005M_harness/M046/S3 ==
  PhyMeasure : Inport
  SensorOut : Outport
  wires:
  PhyMeasure/1 -> SensorOut/1

== system c00005M_harness/M046/S4 ==
  PhyMeasure : Inport
  SensorOut : Outport
  wires:
  PhyMeasure/1 -> SensorOut/1

== system c00005M_harness/M048/Cyber ==
  note: Sensors
  note: Inputs For Window1
  note: Inputs for Window 2
  note: Inputs for window 3
  note: Inputs for window 4
  note: Users
  note: Users
  note: Sensors
  note: Users
  note: Sensors
  note: Users
  note: Sensors
  note: USERS
      | ---------------------------------
      | 0: None
      | 1: Ventana Arriba
      | 2: Ventana hasta arriba
      | 3: Ventana abajo
      | 4: Ventana hasta abajo
  note: 1: SUBE
      | 0: PARADO
      | -1 BAJA
  note: D = Driver (W1)
      | P1 = Passenger 1 (W2)
      | P2 = Passenger 2 (W3)
      | P3 = Passenger 3 (W4)
      | O = Obstacle
      | C = Control
      | Pri = Prioritizer
      | LD = LockDriver
      | PosW = PositionWindow
      | WL = WindowLogic
      | OW = ObstacleWindow
      | CWXC = ControlWindowXCentralized
      | S = Sensor
      | L = Lock
      | WPos = WindowPosition
      | M = Memory
      | InW = InputWindow
      | WIn = WindowInput
  PosW1 : Inport
  PosW2 : Inport  Port=2
  PosW3 : Inport  Port=3
  PosW4 : Inport  Port=4
  DW1 : Inport  Port=5
  DW3 : Inport  Port=6
  DW4 : Inport  Port=7
  P1W2 : Inport  Port=8
  P2W3 : Inport  Port=9
  P1W3 : Inport  Port=10
  P3W4 : Inport  Port=11
  OW1 : Inport  Port=12
  OW2 : Inport  Port=13
  OW3 : Inport  Port=14
  OW4 : Inport  Port=15
  LD : Inport  Port=16
  CW1C : Inport  Port=17
  CW2C : Inport  Port=18
  CW3C : Inport  Port=19
  CW4C : Inport  Port=20
  Pri : Subsystem
  Pri1 : Subsystem
  Pri3 : Subsystem
  Pri4 : Subsystem
  WL : Subsystem
  WL1 : Subsystem
  WL2 : Subsystem
  WL3 : Subsystem
  W1 : Outport
  W2 : Outport  Port=2
  W3 : Outport  Port=3
  W4 : Outport  Port=4
  wires:
  CW4C/1 -> Pri4/3(CW4C)
  CW3C/1 -> Pri1/4(CW3C)
  CW2C/1 -> Pri/2(CW2C)
  CW1C/1 -> Pri3/2(CW1C)
  Pri3/1(User) -> WL/2(User)
  WL3/1(WindowLogicOutput) -> W4/1
  WL2/1(WindowLogicOutput) -> W3/1
  Pri4/1(User) -> WL3/2(User)
  OW4/1 -> WL3/3(OW)
  PosW4/1 -> WL3/1(WPos)
  P3W4/1 -> Pri4/2(P)
  DW4/1 -> Pri4/1(D)
  P1W3/1 -> Pri1/3(P1)
  P2W3/1 -> Pri1/2(P)
  DW3/1 -> Pri1/1(D)
  OW3/1 -> WL2/3(OW)
  PosW3/1 -> WL2/1(WPos)
  Pri1/1(User) -> WL2/2(User)
  WL1/1(WindowLogicOutput) -> W2/1
  OW2/1 -> WL1/3(OW)
  PosW2/1 -> WL1/1(WPos)
  P1W2/1 -> Pri/1(P)
  Pri/1(User) -> WL1/2(User)
  WL/1(WindowLogicOutput) -> W1/1
  DW1/1 -> Pri3/1(D)
  OW1/1 -> WL/3(OW)
  PosW1/1 -> WL/1(WPos)
  LD/1 -> WL3/4(L)

== system c00005M_harness/M048/Physical ==
  InW1 : Inport
  InW2 : Inport  Port=2
  InW3 : Inport  Port=3
  InW4 : Inport  Port=4
  W : Subsystem
  W5 : Subsystem
  W6 : Subsystem
  W7 : Subsystem
  W1 : Outport
  W2 : Outport  Port=2
  W3 : Outport  Port=3
  W4 : Outport  Port=4
  wires:
  W7/1(WPos) -> W4/1
  W6/1(WPos) -> W3/1
  W5/1(WPos) -> W2/1
  W/1(WPos) -> W1/1
  InW4/1 -> W7/1(WIn)
  InW3/1 -> W6/1(WIn)
  InW2/1 -> W5/1(WIn)
  InW1/1 -> W/1(WIn)

== system c00005M_harness/M048/S1 ==
  PhyMeasure : Inport
  SensorOut : Outport
  wires:
  PhyMeasure/1 -> SensorOut/1

== system c00005M_harness/M048/S2 ==
  PhyMeasure : Inport
  SensorOut : Outport
  wires:
  PhyMeasure/1 -> SensorOut/1

== system c00005M_harness/M048/S3 ==
  PhyMeasure : Inport
  SensorOut : Outport
  wires:
  PhyMeasure/1 -> SensorOut/1

== system c00005M_harness/M048/S4 ==
  PhyMeasure : Inport
  SensorOut : Outport
  wires:
  PhyMeasure/1 -> SensorOut/1

== system c00005M_harness/M057/Cyber ==
  note: Sensors
  note: Inputs For Window1
  note: Inputs for Window 2
  note: Inputs for window 3
  note: Inputs for window 4
  note: Users
  note: Users
  note: Sensors
  note: Users
  note: Sensors
  note: Users
  note: Sensors
  note: USERS
      | ---------------------------------
      | 0: None
      | 1: Ventana Arriba
      | 2: Ventana hasta arriba
      | 3: Ventana abajo
      | 4: Ventana hasta abajo
  note: 1: SUBE
      | 0: PARADO
      | -1 BAJA
  note: D = Driver (W1)
      | P1 = Passenger 1 (W2)
      | P2 = Passenger 2 (W3)
      | P3 = Passenger 3 (W4)
      | O = Obstacle
      | C = Control
      | Pri = Prioritizer
      | LD = LockDriver
      | PosW = PositionWindow
      | WL = WindowLogic
      | OW = ObstacleWindow
      | CWXC = ControlWindowXCentralized
      | S = Sensor
      | L = Lock
      | WPos = WindowPosition
      | M = Memory
      | InW = InputWindow
      | WIn = WindowInput
  PosW1 : Inport
  PosW2 : Inport  Port=2
  PosW3 : Inport  Port=3
  PosW4 : Inport  Port=4
  DW1 : Inport  Port=5
  DW3 : Inport  Port=6
  DW4 : Inport  Port=7
  P1W2 : Inport  Port=8
  P2W3 : Inport  Port=9
  P1W3 : Inport  Port=10
  P3W4 : Inport  Port=11
  OW1 : Inport  Port=12
  OW2 : Inport  Port=13
  OW3 : Inport  Port=14
  OW4 : Inport  Port=15
  LD : Inport  Port=16
  CW1C : Inport  Port=17
  CW2C : Inport  Port=18
  CW3C : Inport  Port=19
  CW4C : Inport  Port=20
  Pri : Subsystem
  Pri1 : Subsystem
  Pri3 : Subsystem
  Pri4 : Subsystem
  WL : Subsystem
  WL1 : Subsystem
  WL2 : Subsystem
  WL3 : Subsystem
  W1 : Outport
  W2 : Outport  Port=2
  W3 : Outport  Port=3
  W4 : Outport  Port=4
  wires:
  CW4C/1 -> Pri4/3(CW4C)
  CW3C/1 -> Pri1/4(CW3C)
  CW2C/1 -> Pri/2(CW2C)
  CW1C/1 -> Pri3/2(CW1C)
  Pri3/1(User) -> WL/2(User)
  WL3/1(WindowLogicOutput) -> W4/1
  WL2/1(WindowLogicOutput) -> W3/1
  Pri4/1(User) -> WL3/2(User)
  OW4/1 -> WL3/3(OW)
  PosW4/1 -> WL3/1(WPos)
  P3W4/1 -> Pri4/2(P)
  DW4/1 -> Pri4/1(D)
  P1W3/1 -> Pri1/3(P1)
  P2W3/1 -> Pri1/2(P)
  DW3/1 -> Pri1/1(D)
  OW3/1 -> WL2/3(OW)
  PosW3/1 -> WL2/1(WPos)
  Pri1/1(User) -> WL2/2(User)
  WL1/1(WindowLogicOutput) -> W2/1
  OW2/1 -> WL1/3(OW)
  PosW2/1 -> WL1/1(WPos)
  P1W2/1 -> Pri/1(P)
  Pri/1(User) -> WL1/2(User)
  WL/1(WindowLogicOutput) -> W1/1
  DW1/1 -> Pri3/1(D)
  OW1/1 -> WL/3(OW)
  PosW1/1 -> WL/1(WPos)
  LD/1 -> WL3/4(L)

== system c00005M_harness/M057/Physical ==
  InW1 : Inport
  InW2 : Inport  Port=2
  InW3 : Inport  Port=3
  InW4 : Inport  Port=4
  W : Subsystem
  W5 : Subsystem
  W6 : Subsystem
  W7 : Subsystem
  W1 : Outport
  W2 : Outport  Port=2
  W3 : Outport  Port=3
  W4 : Outport  Port=4
  wires:
  W7/1(WPos) -> W4/1
  W6/1(WPos) -> W3/1
  W5/1(WPos) -> W2/1
  W/1(WPos) -> W1/1
  InW4/1 -> W7/1(WIn)
  InW3/1 -> W6/1(WIn)
  InW2/1 -> W5/1(WIn)
  InW1/1 -> W/1(WIn)

== system c00005M_harness/M057/S1 ==
  PhyMeasure : Inport
  SensorOut : Outport
  wires:
  PhyMeasure/1 -> SensorOut/1

== system c00005M_harness/M057/S2 ==
  PhyMeasure : Inport
  SensorOut : Outport
  wires:
  PhyMeasure/1 -> SensorOut/1

== system c00005M_harness/M057/S3 ==
  PhyMeasure : Inport
  SensorOut : Outport
  wires:
  PhyMeasure/1 -> SensorOut/1

== system c00005M_harness/M057/S4 ==
  PhyMeasure : Inport
  SensorOut : Outport
  wires:
  PhyMeasure/1 -> SensorOut/1

== system c00005M_harness/M058/Cyber ==
  note: Sensors
  note: Inputs For Window1
  note: Inputs for Window 2
  note: Inputs for window 3
  note: Inputs for window 4
  note: Users
  note: Users
  note: Sensors
  note: Users
  note: Sensors
  note: Users
  note: Sensors
  note: USERS
      | ---------------------------------
      | 0: None
      | 1: Ventana Arriba
      | 2: Ventana hasta arriba
      | 3: Ventana abajo
      | 4: Ventana hasta abajo
  note: 1: SUBE
      | 0: PARADO
      | -1 BAJA
  note: D = Driver (W1)
      | P1 = Passenger 1 (W2)
      | P2 = Passenger 2 (W3)
      | P3 = Passenger 3 (W4)
      | O = Obstacle
      | C = Control
      | Pri = Prioritizer
      | LD = LockDriver
      | PosW = PositionWindow
      | WL = WindowLogic
      | OW = ObstacleWindow
      | CWXC = ControlWindowXCentralized
      | S = Sensor
      | L = Lock
      | WPos = WindowPosition
      | M = Memory
      | InW = InputWindow
      | WIn = WindowInput
  PosW1 : Inport
  PosW2 : Inport  Port=2
  PosW3 : Inport  Port=3
  PosW4 : Inport  Port=4
  DW1 : Inport  Port=5
  DW3 : Inport  Port=6
  DW4 : Inport  Port=7
  P1W2 : Inport  Port=8
  P2W3 : Inport  Port=9
  P1W3 : Inport  Port=10
  P3W4 : Inport  Port=11
  OW1 : Inport  Port=12
  OW2 : Inport  Port=13
  OW3 : Inport  Port=14
  OW4 : Inport  Port=15
  LD : Inport  Port=16
  CW1C : Inport  Port=17
  CW2C : Inport  Port=18
  CW3C : Inport  Port=19
  CW4C : Inport  Port=20
  Pri : Subsystem
  Pri1 : Subsystem
  Pri3 : Subsystem
  Pri4 : Subsystem
  WL : Subsystem
  WL1 : Subsystem
  WL2 : Subsystem
  WL3 : Subsystem
  W1 : Outport
  W2 : Outport  Port=2
  W3 : Outport  Port=3
  W4 : Outport  Port=4
  wires:
  CW4C/1 -> Pri4/3(CW4C)
  CW3C/1 -> Pri1/4(CW3C)
  CW2C/1 -> Pri/2(CW2C)
  CW1C/1 -> Pri3/2(CW1C)
  Pri3/1(User) -> WL/2(User)
  WL3/1(WindowLogicOutput) -> W4/1
  WL2/1(WindowLogicOutput) -> W3/1
  Pri4/1(User) -> WL3/2(User)
  OW4/1 -> WL3/3(OW)
  PosW4/1 -> WL3/1(WPos)
  P3W4/1 -> Pri4/2(P)
  DW4/1 -> Pri4/1(D)
  P1W3/1 -> Pri1/3(P1)
  P2W3/1 -> Pri1/2(P)
  DW3/1 -> Pri1/1(D)
  OW3/1 -> WL2/3(OW)
  PosW3/1 -> WL2/1(WPos)
  Pri1/1(User) -> WL2/2(User)
  WL1/1(WindowLogicOutput) -> W2/1
  OW2/1 -> WL1/3(OW)
  PosW2/1 -> WL1/1(WPos)
  P1W2/1 -> Pri/1(P)
  Pri/1(User) -> WL1/2(User)
  WL/1(WindowLogicOutput) -> W1/1
  DW1/1 -> Pri3/1(D)
  OW1/1 -> WL/3(OW)
  PosW1/1 -> WL/1(WPos)
  LD/1 -> WL3/4(L)

== system c00005M_harness/M058/Physical ==
  InW1 : Inport
  InW2 : Inport  Port=2
  InW3 : Inport  Port=3
  InW4 : Inport  Port=4
  W : Subsystem
  W5 : Subsystem
  W6 : Subsystem
  W7 : Subsystem
  W1 : Outport
  W2 : Outport  Port=2
  W3 : Outport  Port=3
  W4 : Outport  Port=4
  wires:
  W7/1(WPos) -> W4/1
  W6/1(WPos) -> W3/1
  W5/1(WPos) -> W2/1
  W/1(WPos) -> W1/1
  InW4/1 -> W7/1(WIn)
  InW3/1 -> W6/1(WIn)
  InW2/1 -> W5/1(WIn)
  InW1/1 -> W/1(WIn)

== system c00005M_harness/M058/S1 ==
  PhyMeasure : Inport
  SensorOut : Outport
  wires:
  PhyMeasure/1 -> SensorOut/1

== system c00005M_harness/M058/S2 ==
  PhyMeasure : Inport
  SensorOut : Outport
  wires:
  PhyMeasure/1 -> SensorOut/1

== system c00005M_harness/M058/S3 ==
  PhyMeasure : Inport
  SensorOut : Outport
  wires:
  PhyMeasure/1 -> SensorOut/1

== system c00005M_harness/M058/S4 ==
  PhyMeasure : Inport
  SensorOut : Outport
  wires:
  PhyMeasure/1 -> SensorOut/1

== system c00005M_harness/CPSUT/Cyber/Pri ==
  P : Inport
  CW2C : Inport  Port=2
  Switch1 : Switch  Criteria=u2 ~= 0
  User : Outport
  wires:
  P/1 -> Switch1/2, Switch1/1
  CW2C/1 -> Switch1/3
  Switch1/1 -> User/1

== system c00005M_harness/CPSUT/Cyber/Pri1 ==
  D : Inport
  P : Inport  Port=2
  P1 : Inport  Port=3
  CW3C : Inport  Port=4
  Switch : Switch  Criteria=u2 ~= 0
  Switch1 : Switch  Criteria=u2 ~= 0
  Switch2 : Switch  Criteria=u2 ~= 0
  User : Outport
  wires:
  Switch/1 -> User/1
  P/1 -> Switch1/1, Switch1/2
  D/1 -> Switch/1, Switch/2
  P1/1 -> Switch2/2, Switch2/1
  Switch1/1 -> Switch/3
  Switch2/1 -> Switch1/3
  CW3C/1 -> Switch2/3

== system c00005M_harness/CPSUT/Cyber/Pri3 ==
  D : Inport
  CW1C : Inport  Port=2
  Switch : Switch  Criteria=u2 ~= 0
  User : Outport
  wires:
  CW1C/1 -> Switch/3
  Switch/1 -> User/1
  D/1 -> Switch/2, Switch/1

== system c00005M_harness/CPSUT/Cyber/Pri4 ==
  D : Inport
  P : Inport  Port=2
  CW4C : Inport  Port=3
  Switch : Switch  Criteria=u2 ~= 0
  Switch1 : Switch  Criteria=u2 ~= 0
  User : Outport
  wires:
  Switch1/1 -> Switch/3
  D/1 -> Switch/2, Switch/1
  P/1 -> Switch1/2, Switch1/1
  Switch/1 -> User/1
  CW4C/1 -> Switch1/3

== system c00005M_harness/CPSUT/Cyber/WL ==
  note: Sensors
  WPos : Inport
  User : Inport  Port=2
  OW : Inport  Port=3
  Chart : Stateflow chart  TreatAsAtomicUnit=on
  Constant : Constant  Value=-1
  Data Type Conversion : DataTypeConversion
  Switch : Switch  Criteria=u2 ~= 0  Threshold=1  ZeroCross=off
  WindowLogicOutput : Outport
  wires:
  OW/1 -> Data Type Conversion/1
  Switch/1 -> WindowLogicOutput/1
  WPos/1 -> Chart/1(S)
  User/1 -> Chart/2(UI)
  Constant/1 -> Switch/1
  Data Type Conversion/1 -> Switch/2
  Chart/1(W) -> Switch/3

== system c00005M_harness/CPSUT/Cyber/WL1 ==
  note: Sensors
  WPos : Inport
  User : Inport  Port=2
  OW : Inport  Port=3
  Chart1 : Stateflow chart  TreatAsAtomicUnit=on
  Constant : Constant  Value=-1
  Data Type Conversion : DataTypeConversion
  Switch : Switch  Criteria=u2 ~= 0  Threshold=1  ZeroCross=off
  WindowLogicOutput : Outport
  wires:
  Data Type Conversion/1 -> Switch/2
  Constant/1 -> Switch/1
  User/1 -> Chart1/2(UI)
  WPos/1 -> Chart1/1(S)
  Switch/1 -> WindowLogicOutput/1
  OW/1 -> Data Type Conversion/1
  Chart1/1(W) -> Switch/3

== system c00005M_harness/CPSUT/Cyber/WL2 ==
  note: Sensors
  WPos : Inport
  User : Inport  Port=2
  OW : Inport  Port=3
  Chart1 : Stateflow chart  TreatAsAtomicUnit=on
  Constant : Constant  Value=-1
  Constant2 : Constant  Value=PosMinimaW3
  Data Type Conversion : DataTypeConversion
  Switch : Switch  Criteria=u2 ~= 0  Threshold=1  ZeroCross=off
  WindowLogicOutput : Outport
  wires:
  OW/1 -> Data Type Conversion/1
  Switch/1 -> WindowLogicOutput/1
  WPos/1 -> Chart1/1(S)
  User/1 -> Chart1/2(UI)
  Constant/1 -> Switch/1
  Data Type Conversion/1 -> Switch/2
  Constant2/1 -> Chart1/3(PosMinW3)
  Chart1/1(W) -> Switch/3

== system c00005M_harness/CPSUT/Cyber/WL3 ==
  note: Sensors
  WPos : Inport
  User : Inport  Port=2
  OW : Inport  Port=3
  L : Inport  Port=4
  Chart2 : Stateflow chart  TreatAsAtomicUnit=on
  Constant : Constant  Value=-1
  Constant1 : Constant  Value=0
  Constant2 : Constant  Value=PosMinimaW4
  Data Type Conversion : DataTypeConversion
  Switch : Switch  Criteria=u2 ~= 0  Threshold=1  ZeroCross=off
  Switch1 : Switch  Criteria=u2 ~= 0
  WindowLogicOutput : Outport
  wires:
  L/1 -> Switch1/2
  Data Type Conversion/1 -> Switch/2
  Constant/1 -> Switch/1
  Chart2/1(W) -> Switch1/3
  User/1 -> Chart2/2(UI)
  WPos/1 -> Chart2/1(S)
  Switch1/1 -> Switch/3
  Constant1/1 -> Switch1/1
  Switch/1 -> WindowLogicOutput/1
  OW/1 -> Data Type Conversion/1
  Constant2/1 -> Chart2/3(PosMinW4)

== system c00005M_harness/CPSUT/Physical/W ==
  WIn : Inport
  DC_Engine : Subsystem
  Discrete-Time Integrator : DiscreteIntegrator  InitialCondition=5  SampleTime=-1  LimitOutput=on  UpperSaturationLimit=5  LowerSaturationLimit=0  ICPrevOutput=DiscIntNeverNeededParam  ICPrevScaledInput=DiscIntNeverNeededParam
  WPos : Outport
  wires:
  Discrete-Time Integrator/1 -> WPos/1
  DC_Engine/1(Speed) -> Discrete-Time Integrator/1
  WIn/1 -> DC_Engine/1(input)

== system c00005M_harness/CPSUT/Physical/W5 ==
  WIn : Inport
  DC_Engine : Subsystem
  Discrete-Time Integrator : DiscreteIntegrator  InitialCondition=5  SampleTime=-1  LimitOutput=on  UpperSaturationLimit=5  LowerSaturationLimit=0  ICPrevOutput=DiscIntNeverNeededParam  ICPrevScaledInput=DiscIntNeverNeededParam
  WPos : Outport
  wires:
  WIn/1 -> DC_Engine/1(input)
  DC_Engine/1(Speed) -> Discrete-Time Integrator/1
  Discrete-Time Integrator/1 -> WPos/1

== system c00005M_harness/CPSUT/Physical/W6 ==
  WIn : Inport
  DC_Engine : Subsystem
  Discrete-Time Integrator : DiscreteIntegrator  InitialCondition=5  SampleTime=-1  LimitOutput=on  UpperSaturationLimit=5  LowerSaturationLimit=PosMinimaW3  ICPrevOutput=DiscIntNeverNeededParam  ICPrevScaledInput=DiscIntNeverNeededParam
  WPos : Outport
  wires:
  Discrete-Time Integrator/1 -> WPos/1
  DC_Engine/1(Speed) -> Discrete-Time Integrator/1
  WIn/1 -> DC_Engine/1(input)

== system c00005M_harness/CPSUT/Physical/W7 ==
  WIn : Inport
  DC_Engine : Subsystem
  Discrete-Time Integrator : DiscreteIntegrator  InitialCondition=5  SampleTime=-1  LimitOutput=on  UpperSaturationLimit=5  LowerSaturationLimit=PosMinimaW4  ICPrevOutput=DiscIntNeverNeededParam  ICPrevScaledInput=DiscIntNeverNeededParam
  WPos : Outport
  wires:
  WIn/1 -> DC_Engine/1(input)
  DC_Engine/1(Speed) -> Discrete-Time Integrator/1
  Discrete-Time Integrator/1 -> WPos/1

== system c00005M_harness/M004/Cyber/Pri ==
  P : Inport
  CW2C : Inport  Port=2
  Switch1 : Switch  Criteria=u2 > Threshold  Threshold=4
  User : Outport
  wires:
  CW2C/1 -> Switch1/3
  P/1 -> Switch1/1, Switch1/2
  Switch1/1 -> User/1

== system c00005M_harness/M004/Cyber/Pri1 ==
  D : Inport
  P : Inport  Port=2
  P1 : Inport  Port=3
  CW3C : Inport  Port=4
  Switch : Switch  Criteria=u2 ~= 0
  Switch1 : Switch  Criteria=u2 ~= 0
  Switch2 : Switch  Criteria=u2 ~= 0
  User : Outport
  wires:
  CW3C/1 -> Switch2/3
  Switch2/1 -> Switch1/3
  Switch1/1 -> Switch/3
  P1/1 -> Switch2/1, Switch2/2
  D/1 -> Switch/2, Switch/1
  P/1 -> Switch1/2, Switch1/1
  Switch/1 -> User/1

== system c00005M_harness/M004/Cyber/Pri3 ==
  D : Inport
  CW1C : Inport  Port=2
  Switch : Switch  Criteria=u2 ~= 0
  User : Outport
  wires:
  D/1 -> Switch/1, Switch/2
  Switch/1 -> User/1
  CW1C/1 -> Switch/3

== system c00005M_harness/M004/Cyber/Pri4 ==
  D : Inport
  P : Inport  Port=2
  CW4C : Inport  Port=3
  Switch : Switch  Criteria=u2 ~= 0
  Switch1 : Switch  Criteria=u2 ~= 0
  User : Outport
  wires:
  Switch/1 -> User/1
  P/1 -> Switch1/1, Switch1/2
  D/1 -> Switch/1, Switch/2
  Switch1/1 -> Switch/3
  CW4C/1 -> Switch1/3

== system c00005M_harness/M004/Cyber/WL ==
  note: Sensors
  WPos : Inport
  User : Inport  Port=2
  OW : Inport  Port=3
  Chart : Stateflow chart  TreatAsAtomicUnit=on
  Constant : Constant  Value=-1
  Data Type Conversion : DataTypeConversion
  Switch : Switch  Criteria=u2 ~= 0  Threshold=1  ZeroCross=off
  WindowLogicOutput : Outport
  wires:
  Data Type Conversion/1 -> Switch/2
  Constant/1 -> Switch/1
  User/1 -> Chart/2(UI)
  WPos/1 -> Chart/1(S)
  Switch/1 -> WindowLogicOutput/1
  OW/1 -> Data Type Conversion/1
  Chart/1(W) -> Switch/3

== system c00005M_harness/M004/Cyber/WL1 ==
  note: Sensors
  WPos : Inport
  User : Inport  Port=2
  OW : Inport  Port=3
  Chart1 : Stateflow chart  TreatAsAtomicUnit=on
  Constant : Constant  Value=-1
  Data Type Conversion : DataTypeConversion
  Switch : Switch  Criteria=u2 ~= 0  Threshold=1  ZeroCross=off
  WindowLogicOutput : Outport
  wires:
  OW/1 -> Data Type Conversion/1
  Switch/1 -> WindowLogicOutput/1
  WPos/1 -> Chart1/1(S)
  User/1 -> Chart1/2(UI)
  Constant/1 -> Switch/1
  Data Type Conversion/1 -> Switch/2
  Chart1/1(W) -> Switch/3

== system c00005M_harness/M004/Cyber/WL2 ==
  note: Sensors
  WPos : Inport
  User : Inport  Port=2
  OW : Inport  Port=3
  Chart1 : Stateflow chart  TreatAsAtomicUnit=on
  Constant : Constant  Value=-1
  Constant2 : Constant  Value=PosMinimaW3
  Data Type Conversion : DataTypeConversion
  Switch : Switch  Criteria=u2 ~= 0  Threshold=1  ZeroCross=off
  WindowLogicOutput : Outport
  wires:
  Constant2/1 -> Chart1/3(PosMinW3)
  Data Type Conversion/1 -> Switch/2
  Constant/1 -> Switch/1
  User/1 -> Chart1/2(UI)
  WPos/1 -> Chart1/1(S)
  Switch/1 -> WindowLogicOutput/1
  OW/1 -> Data Type Conversion/1
  Chart1/1(W) -> Switch/3

== system c00005M_harness/M004/Cyber/WL3 ==
  note: Sensors
  WPos : Inport
  User : Inport  Port=2
  OW : Inport  Port=3
  L : Inport  Port=4
  Chart2 : Stateflow chart  TreatAsAtomicUnit=on
  Constant : Constant  Value=-1
  Constant1 : Constant  Value=0
  Constant2 : Constant  Value=PosMinimaW4
  Data Type Conversion : DataTypeConversion
  Switch : Switch  Criteria=u2 ~= 0  Threshold=1  ZeroCross=off
  Switch1 : Switch  Criteria=u2 ~= 0
  WindowLogicOutput : Outport
  wires:
  Constant2/1 -> Chart2/3(PosMinW4)
  OW/1 -> Data Type Conversion/1
  Switch/1 -> WindowLogicOutput/1
  Constant1/1 -> Switch1/1
  Switch1/1 -> Switch/3
  WPos/1 -> Chart2/1(S)
  User/1 -> Chart2/2(UI)
  Chart2/1(W) -> Switch1/3
  Constant/1 -> Switch/1
  Data Type Conversion/1 -> Switch/2
  L/1 -> Switch1/2

== system c00005M_harness/M004/Physical/W ==
  WIn : Inport
  DC_Engine : Subsystem
  Discrete-Time Integrator : DiscreteIntegrator  InitialCondition=5  SampleTime=-1  LimitOutput=on  UpperSaturationLimit=5  LowerSaturationLimit=0  ICPrevOutput=DiscIntNeverNeededParam  ICPrevScaledInput=DiscIntNeverNeededParam
  WPos : Outport
  wires:
  WIn/1 -> DC_Engine/1(input)
  DC_Engine/1(Speed) -> Discrete-Time Integrator/1
  Discrete-Time Integrator/1 -> WPos/1

== system c00005M_harness/M004/Physical/W5 ==
  WIn : Inport
  DC_Engine : Subsystem
  Discrete-Time Integrator : DiscreteIntegrator  InitialCondition=5  SampleTime=-1  LimitOutput=on  UpperSaturationLimit=5  LowerSaturationLimit=0  ICPrevOutput=DiscIntNeverNeededParam  ICPrevScaledInput=DiscIntNeverNeededParam
  WPos : Outport
  wires:
  Discrete-Time Integrator/1 -> WPos/1
  DC_Engine/1(Speed) -> Discrete-Time Integrator/1
  WIn/1 -> DC_Engine/1(input)

== system c00005M_harness/M004/Physical/W6 ==
  WIn : Inport
  DC_Engine : Subsystem
  Discrete-Time Integrator : DiscreteIntegrator  InitialCondition=5  SampleTime=-1  LimitOutput=on  UpperSaturationLimit=5  LowerSaturationLimit=PosMinimaW3  ICPrevOutput=DiscIntNeverNeededParam  ICPrevScaledInput=DiscIntNeverNeededParam
  WPos : Outport
  wires:
  WIn/1 -> DC_Engine/1(input)
  DC_Engine/1(Speed) -> Discrete-Time Integrator/1
  Discrete-Time Integrator/1 -> WPos/1

== system c00005M_harness/M004/Physical/W7 ==
  WIn : Inport
  DC_Engine : Subsystem
  Discrete-Time Integrator : DiscreteIntegrator  InitialCondition=5  SampleTime=-1  LimitOutput=on  UpperSaturationLimit=5  LowerSaturationLimit=PosMinimaW4  ICPrevOutput=DiscIntNeverNeededParam  ICPrevScaledInput=DiscIntNeverNeededParam
  WPos : Outport
  wires:
  Discrete-Time Integrator/1 -> WPos/1
  DC_Engine/1(Speed) -> Discrete-Time Integrator/1
  WIn/1 -> DC_Engine/1(input)

== system c00005M_harness/M008/Cyber/Pri ==
  P : Inport
  CW2C : Inport  Port=2
  Switch1 : Switch  Criteria=u2 ~= 0
  User : Outport
  wires:
  CW2C/1 -> Switch1/3
  P/1 -> Switch1/1, Switch1/2
  Switch1/1 -> User/1

== system c00005M_harness/M008/Cyber/Pri1 ==
  D : Inport
  P : Inport  Port=2
  P1 : Inport  Port=3
  CW3C : Inport  Port=4
  Switch : Switch  Criteria=u2 > Threshold  Threshold=4
  Switch1 : Switch  Criteria=u2 ~= 0
  Switch2 : Switch  Criteria=u2 ~= 0
  User : Outport
  wires:
  CW3C/1 -> Switch2/3
  Switch2/1 -> Switch1/3
  Switch1/1 -> Switch/3
  P1/1 -> Switch2/1, Switch2/2
  D/1 -> Switch/2, Switch/1
  P/1 -> Switch1/2, Switch1/1
  Switch/1 -> User/1

== system c00005M_harness/M008/Cyber/Pri3 ==
  D : Inport
  CW1C : Inport  Port=2
  Switch : Switch  Criteria=u2 ~= 0
  User : Outport
  wires:
  D/1 -> Switch/1, Switch/2
  Switch/1 -> User/1
  CW1C/1 -> Switch/3

== system c00005M_harness/M008/Cyber/Pri4 ==
  D : Inport
  P : Inport  Port=2
  CW4C : Inport  Port=3
  Switch : Switch  Criteria=u2 ~= 0
  Switch1 : Switch  Criteria=u2 ~= 0
  User : Outport
  wires:
  Switch/1 -> User/1
  P/1 -> Switch1/1, Switch1/2
  D/1 -> Switch/1, Switch/2
  Switch1/1 -> Switch/3
  CW4C/1 -> Switch1/3

== system c00005M_harness/M008/Cyber/WL ==
  note: Sensors
  WPos : Inport
  User : Inport  Port=2
  OW : Inport  Port=3
  Chart : Stateflow chart  TreatAsAtomicUnit=on
  Constant : Constant  Value=-1
  Data Type Conversion : DataTypeConversion
  Switch : Switch  Criteria=u2 ~= 0  Threshold=1  ZeroCross=off
  WindowLogicOutput : Outport
  wires:
  Data Type Conversion/1 -> Switch/2
  Constant/1 -> Switch/1
  User/1 -> Chart/2(UI)
  WPos/1 -> Chart/1(S)
  Switch/1 -> WindowLogicOutput/1
  OW/1 -> Data Type Conversion/1
  Chart/1(W) -> Switch/3

== system c00005M_harness/M008/Cyber/WL1 ==
  note: Sensors
  WPos : Inport
  User : Inport  Port=2
  OW : Inport  Port=3
  Chart1 : Stateflow chart  TreatAsAtomicUnit=on
  Constant : Constant  Value=-1
  Data Type Conversion : DataTypeConversion
  Switch : Switch  Criteria=u2 ~= 0  Threshold=1  ZeroCross=off
  WindowLogicOutput : Outport
  wires:
  OW/1 -> Data Type Conversion/1
  Switch/1 -> WindowLogicOutput/1
  WPos/1 -> Chart1/1(S)
  User/1 -> Chart1/2(UI)
  Constant/1 -> Switch/1
  Data Type Conversion/1 -> Switch/2
  Chart1/1(W) -> Switch/3

== system c00005M_harness/M008/Cyber/WL2 ==
  note: Sensors
  WPos : Inport
  User : Inport  Port=2
  OW : Inport  Port=3
  Chart1 : Stateflow chart  TreatAsAtomicUnit=on
  Constant : Constant  Value=-1
  Constant2 : Constant  Value=PosMinimaW3
  Data Type Conversion : DataTypeConversion
  Switch : Switch  Criteria=u2 ~= 0  Threshold=1  ZeroCross=off
  WindowLogicOutput : Outport
  wires:
  Constant2/1 -> Chart1/3(PosMinW3)
  Data Type Conversion/1 -> Switch/2
  Constant/1 -> Switch/1
  User/1 -> Chart1/2(UI)
  WPos/1 -> Chart1/1(S)
  Switch/1 -> WindowLogicOutput/1
  OW/1 -> Data Type Conversion/1
  Chart1/1(W) -> Switch/3

== system c00005M_harness/M008/Cyber/WL3 ==
  note: Sensors
  WPos : Inport
  User : Inport  Port=2
  OW : Inport  Port=3
  L : Inport  Port=4
  Chart2 : Stateflow chart  TreatAsAtomicUnit=on
  Constant : Constant  Value=-1
  Constant1 : Constant  Value=0
  Constant2 : Constant  Value=PosMinimaW4
  Data Type Conversion : DataTypeConversion
  Switch : Switch  Criteria=u2 ~= 0  Threshold=1  ZeroCross=off
  Switch1 : Switch  Criteria=u2 ~= 0
  WindowLogicOutput : Outport
  wires:
  Constant2/1 -> Chart2/3(PosMinW4)
  OW/1 -> Data Type Conversion/1
  Switch/1 -> WindowLogicOutput/1
  Constant1/1 -> Switch1/1
  Switch1/1 -> Switch/3
  WPos/1 -> Chart2/1(S)
  User/1 -> Chart2/2(UI)
  Chart2/1(W) -> Switch1/3
  Constant/1 -> Switch/1
  Data Type Conversion/1 -> Switch/2
  L/1 -> Switch1/2
